simulink model "three_axis_attitude_control_system"  (R2023a)
settings: Solver=ode5  StartTime=0.0  StopTime=500  FixedStep=0.008  RelTol=1e-3  EnableMultiTasking=on
settings Model: Creator=santhosh  LastModifiedBy=ganes
settings DataIOCC: LimitDataPoints=on  SaveFormat=Array  SignalLoggingSaveFormat=ModelDataLogs  ReturnWorkspaceOutputs=off
settings OptimizationCC: BlockReduction=off  BooleanDataType=off
settings DebuggingCC: SaveWithParameterizedLinksMsg=none  UnderspecifiedInitializationDetection=Classic  MergeDetectMultiDrivingBlocksExec=none  SignalResolutionControl=TryResolveAllWithWarning  MultiTaskDSMMsg=warning  MultiTaskCondExecSysMsg=none  UnconnectedInputMsg=warning  UnconnectedOutputMsg=warning  UnconnectedLineMsg=warning
settings HardwareCC: TargetUnknown=on
settings ModelReferenceCC: PropagateSignalLabelsOutOfModel=off
settings GRTTargetCC: CombineOutputUpdateFcns=off  GRTInterface=on

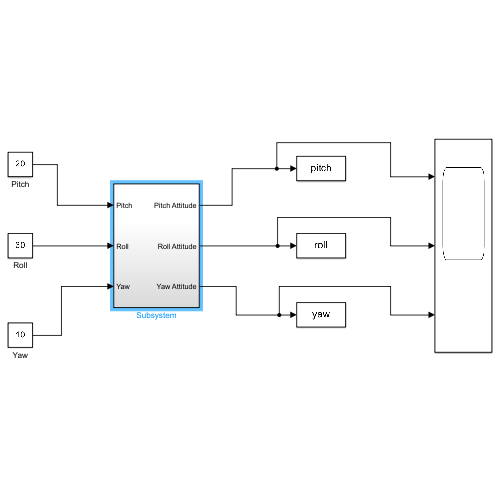
[thumbnail: Simulink's stored preview of the top-level diagram]
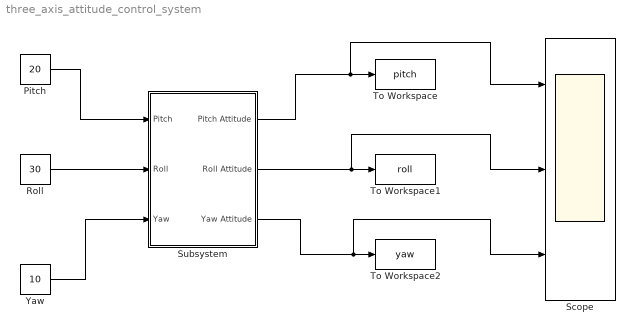
== system three_axis_attitude_control_system ==
  Pitch : Constant  Value=20
  Roll : Constant  Value=30
  Scope : Scope  NumInputPorts=3
  Subsystem : Subsystem
  To Workspace : ToWorkspace  VariableName=pitch  SampleTime=0.008
  To Workspace1 : ToWorkspace  VariableName=roll  SampleTime=0.008
  To Workspace2 : ToWorkspace  VariableName=yaw  SampleTime=0.008
  Yaw : Constant  Value=10
  wires:
  Pitch/1 -> Subsystem/1(Pitch)
  Subsystem/1(Pitch Attitude) -> Scope/1, To Workspace/1
  Subsystem/2(Roll Attitude) -> Scope/2, To Workspace1/1
  Subsystem/3(Yaw Attitude) -> Scope/3, To Workspace2/1
  Roll/1 -> Subsystem/2(Roll)
  Yaw/1 -> Subsystem/3(Yaw)

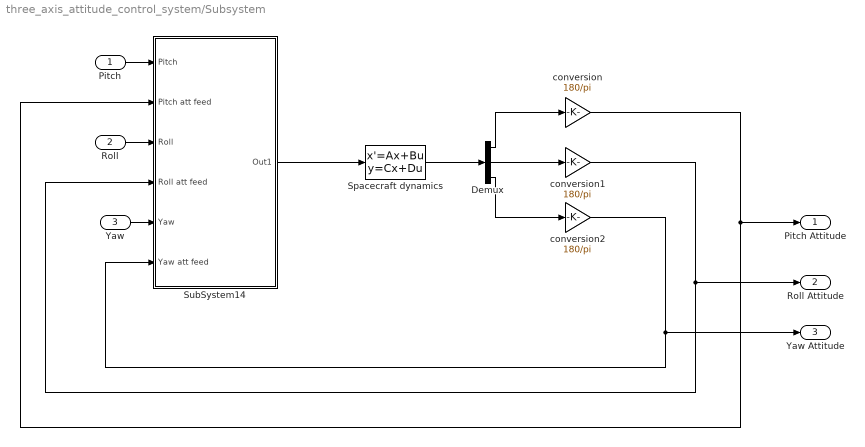
== system three_axis_attitude_control_system/Subsystem ==
  Pitch : Inport
  Roll : Inport  Port=2
  Yaw : Inport  Port=3
  Demux : Demux  Outputs=3
      settings: DisplayOption=none
  Spacecraft dynamics : StateSpace  A=[0 0 0 1 0 0;0 0 0 0 1 0;0 0 0 0 0 1;0 0 0 0 0 0 ;0 0 0 0 0 0;0 0 0 0 0 0]  B=[0 0 0;0 0 0;0 0 0;0.008333 0.0002548 -0.0002317;0.0002548 0.01112 -0.005563;-0.0002317 -0.005563 0.01112]  C=[1 0 0 0 0 0;0 1 0 0 0 0;0 0 1 0 0 0]  D=[0 0 0;0 0 0;0 0 0]  InitialCondition=0
  SubSystem14 : Subsystem
  conversion : Gain  Gain=180/pi  SaturateOnIntegerOverflow=on  OutDataTypeStr=Inherit: Same as input  ParamDataTypeStr=Inherit: Same as input
  conversion1 : Gain  Gain=180/pi  SaturateOnIntegerOverflow=on  OutDataTypeStr=Inherit: Same as input  ParamDataTypeStr=Inherit: Same as input
  conversion2 : Gain  Gain=180/pi  SaturateOnIntegerOverflow=on  OutDataTypeStr=Inherit: Same as input  ParamDataTypeStr=Inherit: Same as input
  Pitch Attitude : Outport
  Roll Attitude : Outport  Port=2
  Yaw Attitude : Outport  Port=3
  wires:
  Spacecraft dynamics/1 -> Demux/1
  SubSystem14/1(Out1) -> Spacecraft dynamics/1
  Pitch/1 -> SubSystem14/1(Pitch)
  Roll/1 -> SubSystem14/3(Roll)
  Yaw/1 -> SubSystem14/5(Yaw)
  Demux/1 -> conversion/1
  conversion2/1 -> SubSystem14/6(Yaw att feed), Yaw Attitude/1
  conversion1/1 -> SubSystem14/4(Roll att feed), Roll Attitude/1
  conversion/1 -> SubSystem14/2(Pitch att feed), Pitch Attitude/1
  Demux/3 -> conversion2/1
  Demux/2 -> conversion1/1

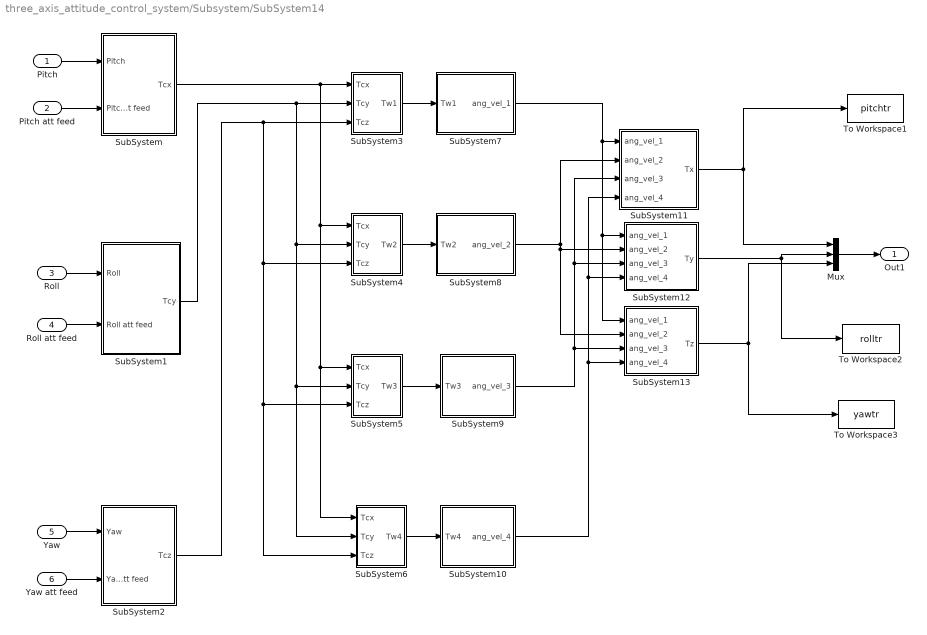
== system three_axis_attitude_control_system/Subsystem/SubSystem14 ==
  Pitch : Inport
  Pitch att feed : Inport  Port=2
  Roll : Inport  Port=3
  Roll att feed : Inport  Port=4
  Yaw : Inport  Port=5
  Yaw att feed : Inport  Port=6
  Mux : Mux  Inputs=3
      settings: DisplayOption=signals
  SubSystem : Subsystem
  SubSystem1 : Subsystem
  SubSystem10 : Subsystem
  SubSystem11 : Subsystem
  SubSystem12 : Subsystem
  SubSystem13 : Subsystem
  SubSystem2 : Subsystem
  SubSystem3 : Subsystem
  SubSystem4 : Subsystem
  SubSystem5 : Subsystem
  SubSystem6 : Subsystem
  SubSystem7 : Subsystem
  SubSystem8 : Subsystem
  SubSystem9 : Subsystem
  To Workspace1 : ToWorkspace  VariableName=pitchtr  SampleTime=0.008
  To Workspace2 : ToWorkspace  VariableName=rolltr  SampleTime=0.008
  To Workspace3 : ToWorkspace  VariableName=yawtr  SampleTime=0.008
  Out1 : Outport
  wires:
  SubSystem7/1(ang_vel_1) -> SubSystem12/1(ang_vel_1), SubSystem13/1(ang_vel_1), SubSystem11/1(ang_vel_1)
  SubSystem8/1(ang_vel_2) -> SubSystem12/2(ang_vel_2), SubSystem13/2(ang_vel_2), SubSystem11/2(ang_vel_2)
  SubSystem9/1(ang_vel_3) -> SubSystem11/3(ang_vel_3), SubSystem12/3(ang_vel_3), SubSystem13/3(ang_vel_3)
  SubSystem10/1(ang_vel_4) -> SubSystem11/4(ang_vel_4), SubSystem12/4(ang_vel_4), SubSystem13/4(ang_vel_4)
  SubSystem11/1(Tx) -> To Workspace1/1, Mux/1
  SubSystem12/1(Ty) -> Mux/2, To Workspace2/1
  SubSystem13/1(Tz) -> Mux/3, To Workspace3/1
  Pitch att feed/1 -> SubSystem/2(Pitch att feed)
  Pitch/1 -> SubSystem/1(Pitch)
  Roll/1 -> SubSystem1/1("Roll ")
  Roll att feed/1 -> SubSystem1/2(Roll att feed)
  Yaw/1 -> SubSystem2/1(Yaw)
  Yaw att feed/1 -> SubSystem2/2(Yaw att feed)
  Mux/1 -> Out1/1
  SubSystem/1(Tcx) -> SubSystem3/1(Tcx), SubSystem4/1(Tcx), SubSystem5/1(Tcx), SubSystem6/1(Tcx)
  SubSystem1/1(Tcy) -> SubSystem3/2(Tcy), SubSystem4/2(Tcy), SubSystem5/2(Tcy), SubSystem6/2(Tcy)
  SubSystem2/1(Tcz) -> SubSystem3/3(Tcz), SubSystem4/3(Tcz), SubSystem5/3(Tcz), SubSystem6/3(Tcz)
  SubSystem3/1(Tw1) -> SubSystem7/1(Tw1)
  SubSystem4/1(Tw2) -> SubSystem8/1(Tw2)
  SubSystem5/1(Tw3) -> SubSystem9/1(Tw3)
  SubSystem6/1(Tw4) -> SubSystem10/1(Tw4)

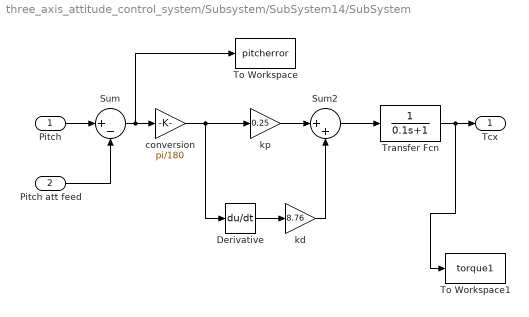
== system three_axis_attitude_control_system/Subsystem/SubSystem14/SubSystem ==
  Pitch : Inport
  Pitch att feed : Inport  Port=2
  Derivative : Derivative
  Sum : Sum  Inputs=|+-  InputSameDT=on  SaturateOnIntegerOverflow=on  OutDataTypeStr=Inherit: Same as first input
  Sum2 : Sum  Inputs=|++  InputSameDT=on  SaturateOnIntegerOverflow=on  OutDataTypeStr=Inherit: Same as first input
  To Workspace : ToWorkspace  VariableName=pitcherror  SampleTime=0.008
  To Workspace1 : ToWorkspace  VariableName=torque1  SampleTime=0.008
  Transfer Fcn : TransferFcn  Denominator=[0.1 1]
  conversion : Gain  Gain=pi/180  SaturateOnIntegerOverflow=on  OutDataTypeStr=Inherit: Same as input  ParamDataTypeStr=Inherit: Same as input
  kd : Gain  Gain=8.76  SaturateOnIntegerOverflow=on  OutDataTypeStr=Inherit: Same as input  ParamDataTypeStr=Inherit: Same as input
  kp : Gain  Gain=0.25  SaturateOnIntegerOverflow=on  OutDataTypeStr=Inherit: Same as input  ParamDataTypeStr=Inherit: Same as input
  Tcx : Outport
  wires:
  Pitch/1 -> Sum/1
  kp/1 -> Sum2/1
  Pitch att feed/1 -> Sum/2
  Sum2/1 -> Transfer Fcn/1
  Transfer Fcn/1 -> Tcx/1, To Workspace1/1
  Sum/1 -> conversion/1, To Workspace/1
  conversion/1 -> kp/1, Derivative/1
  Derivative/1 -> kd/1
  kd/1 -> Sum2/2

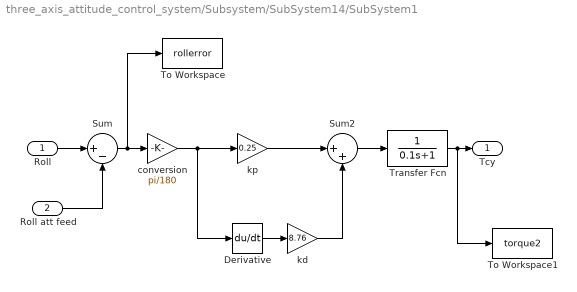
== system three_axis_attitude_control_system/Subsystem/SubSystem14/SubSystem1 ==
  "Roll " : Inport
  Roll att feed : Inport  Port=2
  Derivative : Derivative
  Sum : Sum  Inputs=|+-  InputSameDT=on  SaturateOnIntegerOverflow=on  OutDataTypeStr=Inherit: Same as first input
  Sum2 : Sum  Inputs=|++  InputSameDT=on  SaturateOnIntegerOverflow=on  OutDataTypeStr=Inherit: Same as first input
  To Workspace : ToWorkspace  VariableName=rollerror  SampleTime=0.008
  To Workspace1 : ToWorkspace  VariableName=torque2  SampleTime=0.008
  Transfer Fcn : TransferFcn  Denominator=[0.1 1]
  conversion : Gain  Gain=pi/180  SaturateOnIntegerOverflow=on  OutDataTypeStr=Inherit: Same as input  ParamDataTypeStr=Inherit: Same as input
  kd : Gain  Gain=8.76  SaturateOnIntegerOverflow=on  OutDataTypeStr=Inherit: Same as input  ParamDataTypeStr=Inherit: Same as input
  kp : Gain  Gain=0.25  SaturateOnIntegerOverflow=on  OutDataTypeStr=Inherit: Same as input  ParamDataTypeStr=Inherit: Same as input
  Tcy : Outport
  wires:
  "Roll "/1 -> Sum/1
  kp/1 -> Sum2/1
  kd/1 -> Sum2/2
  Roll att feed/1 -> Sum/2
  Sum2/1 -> Transfer Fcn/1
  Transfer Fcn/1 -> Tcy/1, To Workspace1/1
  Sum/1 -> conversion/1, To Workspace/1
  conversion/1 -> kp/1, Derivative/1
  Derivative/1 -> kd/1

== system three_axis_attitude_control_system/Subsystem/SubSystem14/SubSystem10 ==
  Tw4 : Inport
  Integrator : Integrator
  ang_vel_4 : Outport
  wires:
  Tw4/1 -> Integrator/1
  Integrator/1 -> ang_vel_4/1

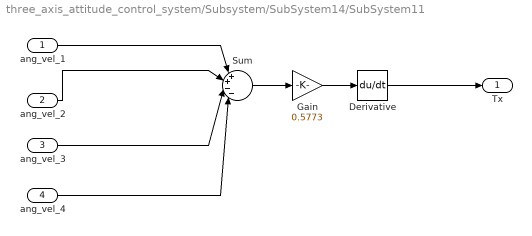
== system three_axis_attitude_control_system/Subsystem/SubSystem14/SubSystem11 ==
  ang_vel_1 : Inport
  ang_vel_2 : Inport  Port=2
  ang_vel_3 : Inport  Port=3
  ang_vel_4 : Inport  Port=4
  Derivative : Derivative
  Gain : Gain  Gain=0.5773  SaturateOnIntegerOverflow=on  OutDataTypeStr=Inherit: Same as input  ParamDataTypeStr=Inherit: Same as input
  Sum : Sum  Inputs=|++--|  InputSameDT=on  SaturateOnIntegerOverflow=on  OutDataTypeStr=Inherit: Same as first input
  Tx : Outport
  wires:
  Sum/1 -> Gain/1
  ang_vel_3/1 -> Sum/3
  ang_vel_2/1 -> Sum/2
  ang_vel_1/1 -> Sum/1
  ang_vel_4/1 -> Sum/4
  Gain/1 -> Derivative/1
  Derivative/1 -> Tx/1

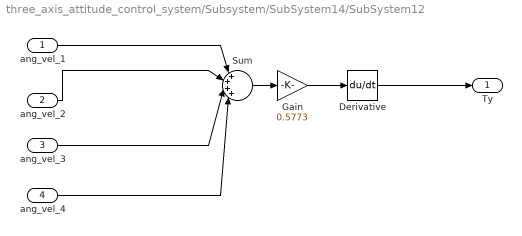
== system three_axis_attitude_control_system/Subsystem/SubSystem14/SubSystem12 ==
  ang_vel_1 : Inport
  ang_vel_2 : Inport  Port=2
  ang_vel_3 : Inport  Port=3
  ang_vel_4 : Inport  Port=4
  Derivative : Derivative
  Gain : Gain  Gain=0.5773  SaturateOnIntegerOverflow=on  OutDataTypeStr=Inherit: Same as input  ParamDataTypeStr=Inherit: Same as input
  Sum : Sum  Inputs=|++++|  InputSameDT=on  SaturateOnIntegerOverflow=on  OutDataTypeStr=Inherit: Same as first input
  Ty : Outport
  wires:
  ang_vel_4/1 -> Sum/4
  ang_vel_1/1 -> Sum/1
  ang_vel_2/1 -> Sum/2
  ang_vel_3/1 -> Sum/3
  Sum/1 -> Gain/1
  Gain/1 -> Derivative/1
  Derivative/1 -> Ty/1

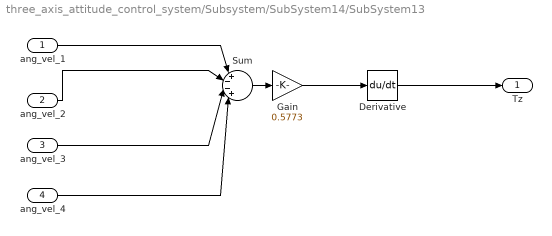
== system three_axis_attitude_control_system/Subsystem/SubSystem14/SubSystem13 ==
  ang_vel_1 : Inport
  ang_vel_2 : Inport  Port=2
  ang_vel_3 : Inport  Port=3
  ang_vel_4 : Inport  Port=4
  Derivative : Derivative
  Gain : Gain  Gain=0.5773  SaturateOnIntegerOverflow=on  OutDataTypeStr=Inherit: Same as input  ParamDataTypeStr=Inherit: Same as input
  Sum : Sum  Inputs=|+--+|  InputSameDT=on  SaturateOnIntegerOverflow=on  OutDataTypeStr=Inherit: Same as first input
  Tz : Outport
  wires:
  Sum/1 -> Gain/1
  ang_vel_3/1 -> Sum/3
  ang_vel_2/1 -> Sum/2
  ang_vel_1/1 -> Sum/1
  ang_vel_4/1 -> Sum/4
  Gain/1 -> Derivative/1
  Derivative/1 -> Tz/1

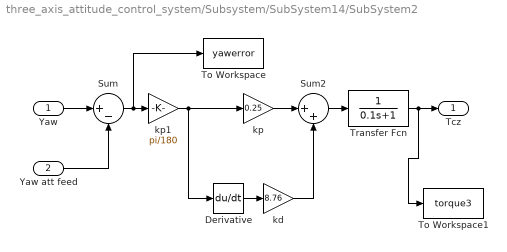
== system three_axis_attitude_control_system/Subsystem/SubSystem14/SubSystem2 ==
  Yaw : Inport
  Yaw att feed : Inport  Port=2
  Derivative : Derivative
  Sum : Sum  Inputs=|+-  InputSameDT=on  SaturateOnIntegerOverflow=on  OutDataTypeStr=Inherit: Same as first input
  Sum2 : Sum  Inputs=|++  InputSameDT=on  SaturateOnIntegerOverflow=on  OutDataTypeStr=Inherit: Same as first input
  To Workspace : ToWorkspace  VariableName=yawerror  SampleTime=0.008
  To Workspace1 : ToWorkspace  VariableName=torque3  SampleTime=0.008
  Transfer Fcn : TransferFcn  Denominator=[0.1 1]
  kd : Gain  Gain=8.76  SaturateOnIntegerOverflow=on  OutDataTypeStr=Inherit: Same as input  ParamDataTypeStr=Inherit: Same as input
  kp : Gain  Gain=0.25  SaturateOnIntegerOverflow=on  OutDataTypeStr=Inherit: Same as input  ParamDataTypeStr=Inherit: Same as input
  kp1 : Gain  Gain=pi/180  SaturateOnIntegerOverflow=on  OutDataTypeStr=Inherit: Same as input  ParamDataTypeStr=Inherit: Same as input
  Tcz : Outport
  wires:
  Yaw/1 -> Sum/1
  Derivative/1 -> kd/1
  kp/1 -> Sum2/1
  kd/1 -> Sum2/2
  Yaw att feed/1 -> Sum/2
  Sum2/1 -> Transfer Fcn/1
  Transfer Fcn/1 -> Tcz/1, To Workspace1/1
  Sum/1 -> kp1/1, To Workspace/1
  kp1/1 -> kp/1, Derivative/1

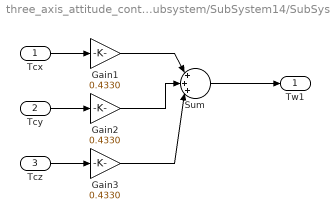
== system three_axis_attitude_control_system/Subsystem/SubSystem14/SubSystem3 ==
  Tcx : Inport
  Tcy : Inport  Port=2
  Tcz : Inport  Port=3
  Gain1 : Gain  Gain=0.4330  SaturateOnIntegerOverflow=on  OutDataTypeStr=Inherit: Same as input  ParamDataTypeStr=Inherit: Same as input
  Gain2 : Gain  Gain=0.4330  SaturateOnIntegerOverflow=on  OutDataTypeStr=Inherit: Same as input  ParamDataTypeStr=Inherit: Same as input
  Gain3 : Gain  Gain=0.4330  SaturateOnIntegerOverflow=on  OutDataTypeStr=Inherit: Same as input  ParamDataTypeStr=Inherit: Same as input
  Sum : Sum  Inputs=|+++|  InputSameDT=on  SaturateOnIntegerOverflow=on  OutDataTypeStr=Inherit: Same as first input
  Tw1 : Outport
  wires:
  Sum/1 -> Tw1/1
  Gain1/1 -> Sum/1
  Tcx/1 -> Gain1/1
  Tcy/1 -> Gain2/1
  Gain2/1 -> Sum/2
  Tcz/1 -> Gain3/1
  Gain3/1 -> Sum/3

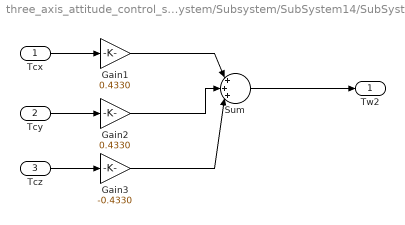
== system three_axis_attitude_control_system/Subsystem/SubSystem14/SubSystem4 ==
  Tcx : Inport
  Tcy : Inport  Port=2
  Tcz : Inport  Port=3
  Gain1 : Gain  Gain=0.4330  SaturateOnIntegerOverflow=on  OutDataTypeStr=Inherit: Same as input  ParamDataTypeStr=Inherit: Same as input
  Gain2 : Gain  Gain=0.4330  OutDataTypeStr=Inherit: Same as input  ParamDataTypeStr=Inherit: Same as input
  Gain3 : Gain  Gain=-0.4330  SaturateOnIntegerOverflow=on  OutDataTypeStr=Inherit: Same as input  ParamDataTypeStr=Inherit: Same as input
  Sum : Sum  Inputs=|+++|  InputSameDT=on  SaturateOnIntegerOverflow=on  OutDataTypeStr=Inherit: Same as first input
  Tw2 : Outport
  wires:
  Sum/1 -> Tw2/1
  Tcz/1 -> Gain3/1
  Gain3/1 -> Sum/3
  Gain2/1 -> Sum/2
  Tcy/1 -> Gain2/1
  Tcx/1 -> Gain1/1
  Gain1/1 -> Sum/1

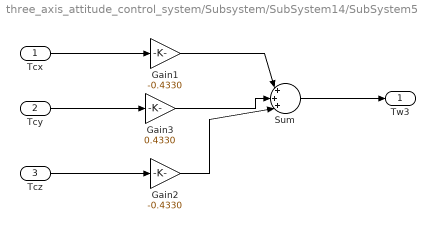
== system three_axis_attitude_control_system/Subsystem/SubSystem14/SubSystem5 ==
  Tcx : Inport
  Tcy : Inport  Port=2
  Tcz : Inport  Port=3
  Gain1 : Gain  Gain=-0.4330  SaturateOnIntegerOverflow=on  OutDataTypeStr=Inherit: Same as input  ParamDataTypeStr=Inherit: Same as input
  Gain2 : Gain  Gain=-0.4330  SaturateOnIntegerOverflow=on  OutDataTypeStr=Inherit: Same as input  ParamDataTypeStr=Inherit: Same as input
  Gain3 : Gain  Gain=0.4330  SaturateOnIntegerOverflow=on  OutDataTypeStr=Inherit: Same as input  ParamDataTypeStr=Inherit: Same as input
  Sum : Sum  Inputs=|+++|  InputSameDT=on  SaturateOnIntegerOverflow=on  OutDataTypeStr=Inherit: Same as first input
  Tw3 : Outport
  wires:
  Sum/1 -> Tw3/1
  Gain3/1 -> Sum/2
  Gain2/1 -> Sum/3
  Tcz/1 -> Gain2/1
  Tcy/1 -> Gain3/1
  Tcx/1 -> Gain1/1
  Gain1/1 -> Sum/1

== system three_axis_attitude_control_system/Subsystem/SubSystem14/SubSystem6 ==
  Tcx : Inport
  Tcy : Inport  Port=2
  Tcz : Inport  Port=3
  Gain1 : Gain  Gain=-0.4330  SaturateOnIntegerOverflow=on  OutDataTypeStr=Inherit: Same as input  ParamDataTypeStr=Inherit: Same as input
  Gain2 : Gain  Gain=0.4330  SaturateOnIntegerOverflow=on  OutDataTypeStr=Inherit: Same as input  ParamDataTypeStr=Inherit: Same as input
  Gain3 : Gain  Gain=0.4330  SaturateOnIntegerOverflow=on  OutDataTypeStr=Inherit: Same as input  ParamDataTypeStr=Inherit: Same as input
  Sum : Sum  Inputs=|+++|  InputSameDT=on  SaturateOnIntegerOverflow=on  OutDataTypeStr=Inherit: Same as first input
  Tw4 : Outport
  wires:
  Sum/1 -> Tw4/1
  Tcz/1 -> Gain3/1
  Gain3/1 -> Sum/3
  Gain2/1 -> Sum/2
  Tcx/1 -> Gain1/1
  Tcy/1 -> Gain2/1
  Gain1/1 -> Sum/1

== system three_axis_attitude_control_system/Subsystem/SubSystem14/SubSystem7 ==
  Tw1 : Inport
  Integrator : Integrator
  ang_vel_1 : Outport
  wires:
  Integrator/1 -> ang_vel_1/1
  Tw1/1 -> Integrator/1

== system three_axis_attitude_control_system/Subsystem/SubSystem14/SubSystem8 ==
  Tw2 : Inport
  Integrator : Integrator
  ang_vel_2 : Outport
  wires:
  Tw2/1 -> Integrator/1
  Integrator/1 -> ang_vel_2/1

== system three_axis_attitude_control_system/Subsystem/SubSystem14/SubSystem9 ==
  Tw3 : Inport
  Integrator : Integrator
  ang_vel_3 : Outport
  wires:
  Integrator/1 -> ang_vel_3/1
  Tw3/1 -> Integrator/1
